simulink subsystem "LW_noaileron_dynamic"  (R2024b)
settings: Solver=VariableStepAuto  StartTime=0.0  StopTime=10.0  RelTol=1e-3
undefined symbols (not defined in the file or in its folder): decyear, DiscIntNeverNeededParam, Earth, F, Light, LW_ANGLE, MIL, ModelFailWind_ConstWindX, ModelFailWind_ConstWindY, ModelFailWind_ConstWindZ, ModelFailWind_GustWindFreq, ModelFailWind_GustWindStrength, ModelFailWind_isConstWind, ModelFailWind_isEnable, ModelFailWind_isGustWind, ModelFailWind_isSheerWind, ModelFailWind_isTurbWind, ModelInit_AngEuler, ModelInit_PosE, ModelInit_Rads, ModelInit_RateB, ModelInit_servoRads, ModelInit_VelB, ModelParam_DeltaRatemax, ModelParam_efficiency, ModelParam_envAltitude, ModelParam_LBb, ModelParam_LBc, ModelParam_LBClp, ModelParam_LBCmq, ModelParam_LBCnr, ModelParam_LBRho, ModelParam_LBS, ModelParam_lDeltamax, ModelParam_lDeltamin, ModelParam_motorp1, ModelParam_motorp2, ModelParam_motorp3, ModelParam_motorT, ModelParam_motorUp1, ModelParam_motorUp2, ModelParam_motorUp3, ModelParam_noiseFBa, ModelParam_noiseFBaSeed, ModelParam_noiseFNa, ModelParam_noiseFNaSeed, ModelParam_noiseMNa, ModelParam_noiseMNaSeed, ModelParam_rDeltamax, ModelParam_rDeltamin, ModelParam_servoT, ModelParam_temperature, ModelParam_uavCCm, ModelParam_uavCd, ModelParam_uavJ, ModelParam_uavMass, ModelParam_use_CoesaAtmosphereModel_density, ModelParam_use_CoesaAtmosphereModel_temperature, ModelReset_Euler, ModelReset_Pos ... (+5)
libraries: simulink x5, aerolibwind2 x3, sharedtransform x2, sharedutil x2, aerolibtransform2 x1, aerolibasang x1, aerolibatmos2 x1, aerolibconvert2 x1, aerolibgravity2 x1, shared6dof x1
(part 1 of 2)
settings Model: Creator=DELL  LastModifiedBy=bhcxq
settings SolverCC: AlgebraicLoopSolver=TrustRegion
settings DebuggingCC: UnconnectedInputMsg=warning  UnconnectedOutputMsg=warning  UnconnectedLineMsg=warning
settings ModelReferenceCC: EnableRefExpFcnMdlSchedulingChecks=on
settings RTWCC: GPUComputeCapability=3.5  DLArmComputeVersion=19.05

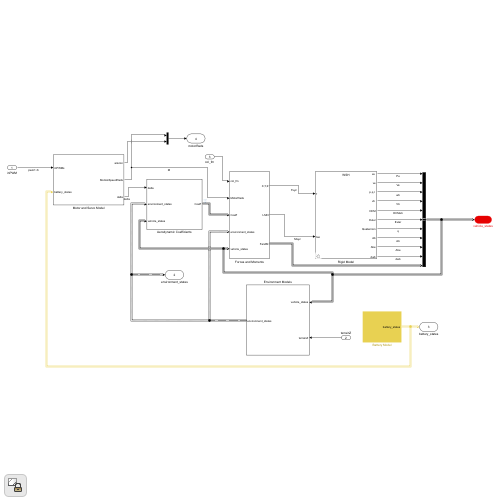
[thumbnail: Simulink's stored preview of the top-level diagram]
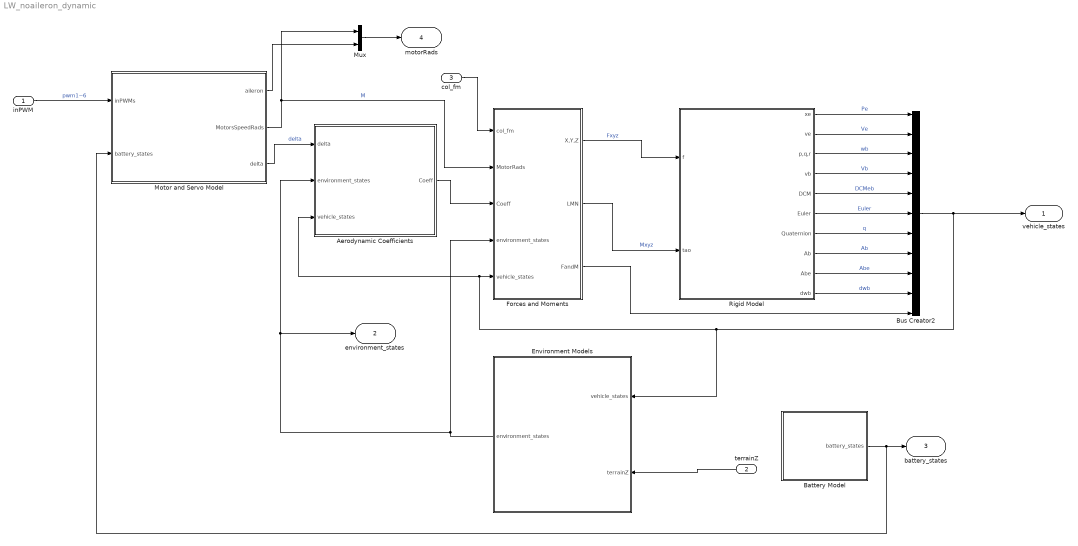
== system LW_noaileron_dynamic ==
  inPWM : Inport
  terrainZ : Inport  Port=2
  col_fm : Inport  Port=3
  Aerodynamic Coefficients : Subsystem
  Battery Model : Subsystem
  Bus Creator2 : BusCreator  Inputs=11
  Environment Models : Subsystem
  Forces and Moments : Subsystem
  Motor and Servo Model : Subsystem
  Mux : Mux  Inputs=2
  Rigid Model : Subsystem  Variant=on
  vehicle_states : Outport
  environment_states : Outport  Port=2
  battery_states : Outport  Port=3
  motorRads : Outport  Port=4
  wires:
  Rigid Model/5(DCM) -> Bus Creator2/5  "DCMeb"
  Rigid Model/9(Abe) -> Bus Creator2/9  "Abe"
  Rigid Model/4("vb ") -> Bus Creator2/4  "Vb"
  Rigid Model/2(ve) -> Bus Creator2/2  "Ve"
  Bus Creator2/1 -> Aerodynamic Coefficients/3(vehicle_states), Forces and Moments/5(vehicle_states), Environment Models/1(vehicle_states), vehicle_states/1
  Forces and Moments/1(X,Y,Z) -> Rigid Model/1(f)  "Fxyz"
  Rigid Model/1("xe ") -> Bus Creator2/1  "Pe"
  Forces and Moments/2(LMN) -> Rigid Model/2(tao)  "Mxyz"
  Rigid Model/6(Euler) -> Bus Creator2/6  "Euler"
  Aerodynamic Coefficients/1(Coeff) -> Forces and Moments/3(Coeff)
  Rigid Model/8(Ab) -> Bus Creator2/8  "Ab"
  inPWM/1 -> Motor and Servo Model/1(inPWMs)  "pwm1~6"
  Environment Models/1(environment_states) -> Aerodynamic Coefficients/2(environment_states), environment_states/1, Forces and Moments/4(environment_states)
  Rigid Model/3("p,q,r ") -> Bus Creator2/3  "wb"
  Motor and Servo Model/2(MotorsSpeedRads) -> Forces and Moments/2(MotorRads), Mux/1  "M"
  Mux/1 -> motorRads/1
  Motor and Servo Model/3(delta) -> Aerodynamic Coefficients/1(delta)  "delta"
  Rigid Model/7(Quaternion) -> Bus Creator2/7  "q"
  Battery Model/1(battery_states) -> battery_states/1, Motor and Servo Model/2(battery_states)
  Rigid Model/10(dwb) -> Bus Creator2/10  "dwb"
  terrainZ/1 -> Environment Models/2(terrainZ)
  Forces and Moments/3(FandM) -> Bus Creator2/11
  col_fm/1 -> Forces and Moments/1(col_fm)
  Motor and Servo Model/1(aileron) -> Mux/2

== system LW_noaileron_dynamic/Aerodynamic Coefficients ==
  delta : Inport
  environment_states : Inport  Port=2
  vehicle_states : Inport  Port=3
  Bus Creator : BusCreator  Inputs=6
  Bus Selector : BusSelector  OutputSignals=alpha,beta,airspeed  OutputAsBus=on
  Bus Selector1 : BusSelector  OutputSignals=wb  OutputAsBus=on
  aerodynamic coefficients : MATLAB Function  TreatAsAtomicUnit=on
  Coeff : Outport  VectorParamsAs1DForOutWhenUnconnected=off
  wires:
  aerodynamic coefficients/8(C_me) -> ?  "C_me"
  aerodynamic coefficients/7(C_m0) -> ?  "C_m0"
  environment_states/1 -> Bus Selector/1
  Bus Creator/1 -> Coeff/1
  aerodynamic coefficients/4(C_l) -> Bus Creator/4  "C_l"
  aerodynamic coefficients/5(C_m) -> Bus Creator/5  "C_m"
  aerodynamic coefficients/6(C_n) -> Bus Creator/6  "C_n"
  delta/1 -> aerodynamic coefficients/3(delta)
  Bus Selector/1 -> aerodynamic coefficients/1(incid)
  vehicle_states/1 -> Bus Selector1/1
  Bus Selector1/1 -> aerodynamic coefficients/2(wb)
  aerodynamic coefficients/1(C_D) -> Bus Creator/1  "C_D"
  aerodynamic coefficients/3(C_L) -> Bus Creator/3  "C_L"
  aerodynamic coefficients/2(C_Y) -> Bus Creator/2  "C_Y"

== system LW_noaileron_dynamic/Battery Model ==
  BatteryVol : Constant  Value=16
  Bus Creator : BusCreator  Inputs=2
  Constant : Constant  Value=4000
  battery_states : Outport
  wires:
  BatteryVol/1 -> Bus Creator/1  "Ub"
  Constant/1 -> Bus Creator/2  "RemCapa"
  Bus Creator/1 -> battery_states/1

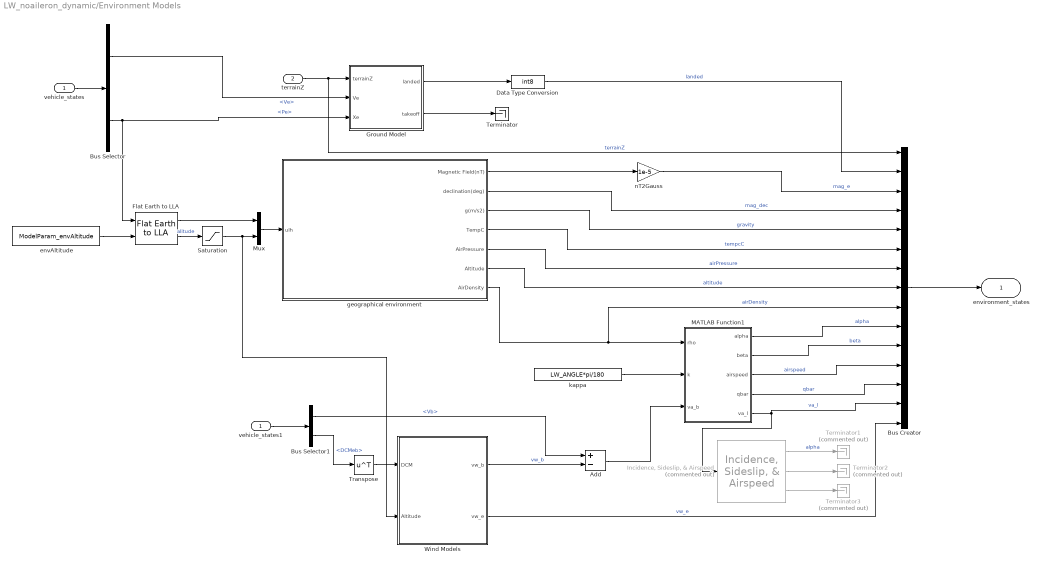
== system LW_noaileron_dynamic/Environment Models ==
  vehicle_states : Inport
  terrainZ : Inport  Port=2
  Add : Sum  Inputs=+-
  Bus Creator : BusCreator  Inputs=15  OutDataTypeStr=Bus: EnvironmentStates  NonVirtualBus=on
  Bus Selector : BusSelector  OutputSignals=Ve,Pe
  Bus Selector1 : BusSelector  OutputSignals=Vb,DCMeb
  Data Type Conversion : DataTypeConversion  OutDataTypeStr=int8  SaturateOnIntegerOverflow=off  RndMeth=Floor
  Flat Earth to LLA : aerolibtransform2/Flat Earth to LLA  units=Metric (MKS)  ptype=Earth (WGS84)  F=1/298.257223563  R=6378137  refPosPort=off  LL0=ModelParam_GPSLatLong  psi=0
  Ground Model : MATLAB Function  TreatAsAtomicUnit=on
  "Incidence, Sideslip, & Airspeed" : aerolibasang/Incidence, Sideslip, & Airspeed  Commented=on
  MATLAB Function1 : MATLAB Function  TreatAsAtomicUnit=on
  Mux : Mux  Inputs=2
  Saturation : Saturate  UpperLimit=10000  LowerLimit=0
  Terminator : Terminator
  Terminator1 : Terminator  Commented=on
  Terminator2 : Terminator  Commented=on
  Terminator3 : Terminator  Commented=on
  Transpose : Math  Operator=transpose  SignedPower=on
  Wind Models : Subsystem  TreatAsAtomicUnit=on
  envAltitude : Constant  Value=ModelParam_envAltitude
  geographical environment : Subsystem
  kappa : Constant  Value=LW_ANGLE*pi/180
  nT2Gauss : Gain  Gain=1e-5
  vehicle_states1 : InportShadow
  environment_states : Outport
  wires:
  MATLAB Function1/1(alpha) -> Bus Creator/10  "alpha"
  "Incidence, Sideslip, & Airspeed"/1 -> Terminator1/1  "alpha"
  "Incidence, Sideslip, & Airspeed"/3 -> Terminator3/1
  "Incidence, Sideslip, & Airspeed"/2 -> Terminator2/1
  MATLAB Function1/5(va_l) -> "Incidence, Sideslip, & Airspeed"/1, Bus Creator/14  "va_l"
  Flat Earth to LLA/2 -> Saturation/1  "alitude"
  vehicle_states/1 -> Bus Selector/1
  Bus Selector1/2 -> Transpose/1  "<DCMeb>"
  geographical environment/3(g(m/s2)) -> Bus Creator/5  "gravity"
  Mux/1 -> geographical environment/1(ulh)
  Flat Earth to LLA/1 -> Mux/1
  envAltitude/1 -> Flat Earth to LLA/2
  Transpose/1 -> Wind Models/1(DCM)
  geographical environment/1(Magnetic Field(nT)) -> nT2Gauss/1
  Bus Selector/2 -> Flat Earth to LLA/1, Ground Model/3(Xe)  "<Pe>"
  nT2Gauss/1 -> Bus Creator/3  "mag_e"
  geographical environment/2(declination(deg)) -> Bus Creator/4  "mag_dec"
  geographical environment/4(TempC) -> Bus Creator/6  "tempcC"
  geographical environment/5(AirPressure) -> Bus Creator/7  "airPressure"
  geographical environment/7(AirDensity) -> MATLAB Function1/1(rho), Bus Creator/9  "airDensity"
  Bus Creator/1 -> environment_states/1
  MATLAB Function1/2(beta) -> Bus Creator/11  "beta"
  MATLAB Function1/4(qbar) -> Bus Creator/13  "qbar"
  MATLAB Function1/3(airspeed) -> Bus Creator/12  "airspeed"
  Wind Models/1(vw_b) -> Add/2  "vw_b"
  kappa/1 -> MATLAB Function1/2(k)
  Bus Selector/1 -> Ground Model/2(Ve)  "<Ve>"
  Ground Model/2(takeoff) -> Terminator/1
  Ground Model/1(landed) -> Data Type Conversion/1
  terrainZ/1 -> Ground Model/1(terrainZ), Bus Creator/1  "terrainZ"
  Data Type Conversion/1 -> Bus Creator/2  "landed"
  Add/1 -> MATLAB Function1/3(va_b)
  Wind Models/2(vw_e) -> Bus Creator/15  "vw_e"
  vehicle_states1/1 -> Bus Selector1/1
  Bus Selector1/1 -> Add/1  "<Vb>"
  geographical environment/6(Altitude) -> Bus Creator/8  "altitude"
  Saturation/1 -> Wind Models/2(Altitude), Mux/2

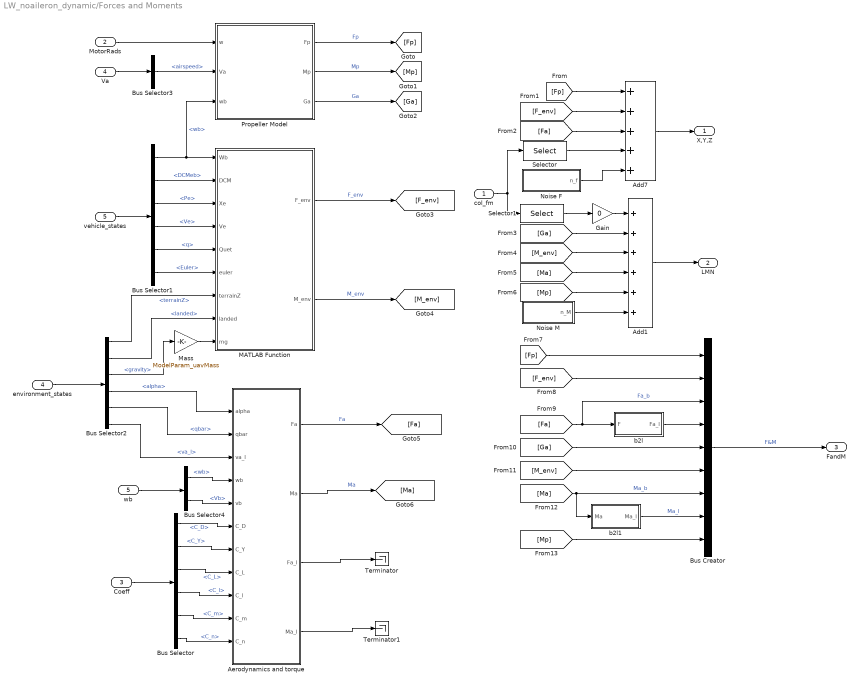
== system LW_noaileron_dynamic/Forces and Moments ==
  col_fm : Inport
  MotorRads : Inport  Port=2
  Coeff : Inport  Port=3
  environment_states : Inport  Port=4
  vehicle_states : Inport  Port=5
  Add1 : Sum  Inputs=++++++
  Add7 : Sum  Inputs=+++++
  Aerodynamics and torque : MATLAB Function  TreatAsAtomicUnit=on
  Bus Creator : BusCreator  Inputs=9
  Bus Selector : BusSelector  OutputSignals=C_D,C_Y,C_L,C_l,C_m,C_n
  Bus Selector1 : BusSelector  OutputSignals=wb,DCMeb,Pe,Ve,q,Euler
  Bus Selector2 : BusSelector  OutputSignals=terrainZ,landed,gravity,alpha,qbar,va_l
  Bus Selector3 : BusSelector  OutputSignals=airspeed
  Bus Selector4 : BusSelector  OutputSignals=wb,Vb
  Gain : Gain  Gain=0
  MATLAB Function : MATLAB Function  TreatAsAtomicUnit=on
  Mass : Gain  Gain=ModelParam_uavMass
  Noise F : Subsystem
  Noise M : Subsystem
  Propeller Model : MATLAB Function  TreatAsAtomicUnit=on
  Selector : Selector  InputPortWidth=6  IndexOptions=Index vector (dialog)  Indices=[1:3]  OutputSizes=1
  Selector1 : Selector  InputPortWidth=6  IndexOptions=Index vector (dialog)  Indices=[4:6]  OutputSizes=1
  Terminator : Terminator
  Terminator1 : Terminator
  Va : InportShadow  Port=4
  b2l : MATLAB Function  TreatAsAtomicUnit=on
  b2l1 : MATLAB Function  TreatAsAtomicUnit=on
  wb : InportShadow  Port=5
  X,Y,Z : Outport  PortDimensions=[3,1]  VectorParamsAs1DForOutWhenUnconnected=off
  LMN : Outport  Port=2  PortDimensions=[3,1]  VectorParamsAs1DForOutWhenUnconnected=off
  FandM : Outport  Port=3  VectorParamsAs1DForOutWhenUnconnected=off
  wires:
  Gain/1 -> Add1/1
  Noise M/1(n_M) -> Add1/6
  Noise F/1(n_f) -> Add7/5
  Aerodynamics and torque/4(Ma_l) -> Terminator1/1
  Aerodynamics and torque/3(Fa_l) -> Terminator/1
  b2l1/1(Ma_l) -> Bus Creator/8  "Ma_l"
  Selector1/1 -> Gain/1
  Selector/1 -> Add7/4
  col_fm/1 -> Selector1/1, Selector/1
  b2l/1(Fa_l) -> Bus Creator/4
  [Mp] -> Bus Creator/9
  [Ma] -> b2l1/1(Ma), Bus Creator/7  "Ma_b"
  [M_env] -> Bus Creator/6
  [Ga] -> Bus Creator/5
  [Fa] -> b2l/1(F), Bus Creator/3  "Fa_b"
  [F_env] -> Bus Creator/2
  [Fp] -> Bus Creator/1
  [Mp] -> Add1/5
  [Ma] -> Add1/4
  [M_env] -> Add1/3
  [Ga] -> Add1/2
  [Fa] -> Add7/3
  [F_env] -> Add7/2
  Aerodynamics and torque/2(Ma) -> [Ma]  "Ma"
  Aerodynamics and torque/1(Fa) -> [Fa]  "Fa"
  MATLAB Function/2(M_env) -> [M_env]  "M_env"
  [Fp] -> Add7/1
  Bus Creator/1 -> FandM/1  "F&M"
  Bus Selector2/2 -> MATLAB Function/8(landed)  "<landed>"
  Bus Selector1/6 -> MATLAB Function/6(euler)  "<Euler>"
  Bus Selector4/1 -> Aerodynamics and torque/4(wb)  "<wb>"
  Bus Selector2/6 -> Aerodynamics and torque/3(va_l)  "<va_l>"
  wb/1 -> Bus Selector4/1
  Bus Selector2/5 -> Aerodynamics and torque/2(qbar)  "<qbar>"
  Propeller Model/1(Fp) -> [Fp]  "Fp"
  Add7/1 -> X,Y,Z/1
  Propeller Model/2(Mp) -> [Mp]  "Mp"
  Add1/1 -> LMN/1
  environment_states/1 -> Bus Selector2/1
  Coeff/1 -> Bus Selector/1
  Bus Selector/1 -> Aerodynamics and torque/6(C_D)  "<C_D>"
  Bus Selector/2 -> Aerodynamics and torque/7(C_Y)  "<C_Y>"
  Bus Selector/3 -> Aerodynamics and torque/8(C_L)  "<C_L>"
  Bus Selector/4 -> Aerodynamics and torque/9(C_l)  "<C_l>"
  Bus Selector/5 -> Aerodynamics and torque/10(C_m)  "<C_m>"
  Bus Selector/6 -> Aerodynamics and torque/11(C_n)  "<C_n>"
  Propeller Model/3(Ga) -> [Ga]  "Ga"
  MotorRads/1 -> Propeller Model/1(w)
  Bus Selector3/1 -> Propeller Model/2(Va)  "<airspeed>"
  Bus Selector1/1 -> Propeller Model/3(wb), MATLAB Function/1(Wb)  "<wb>"
  Bus Selector1/5 -> MATLAB Function/5(Quet)  "<q>"
  Bus Selector1/3 -> MATLAB Function/3(Xe)  "<Pe>"
  Bus Selector2/1 -> MATLAB Function/7(terrainZ)  "<terrainZ>"
  Bus Selector1/2 -> MATLAB Function/2(DCM)  "<DCMeb>"
  MATLAB Function/1(F_env) -> [F_env]  "F_env"
  vehicle_states/1 -> Bus Selector1/1
  Bus Selector1/4 -> MATLAB Function/4(Ve)  "<Ve>"
  Bus Selector2/4 -> Aerodynamics and torque/1(alpha)  "<alpha>"
  Va/1 -> Bus Selector3/1
  Bus Selector2/3 -> Mass/1  "<gravity>"
  Mass/1 -> MATLAB Function/9(mg)
  Bus Selector4/2 -> Aerodynamics and torque/5(vb)  "<Vb>"

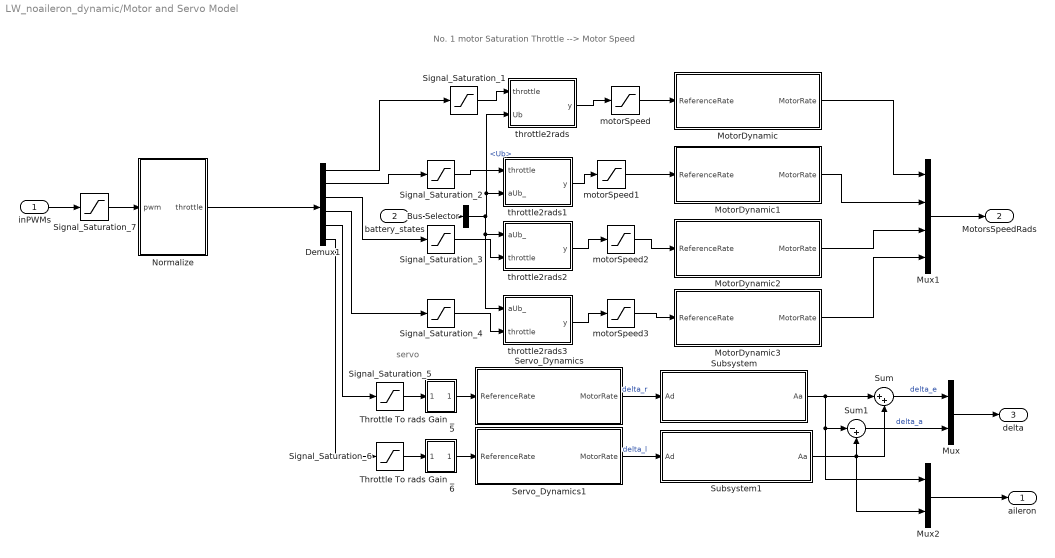
== system LW_noaileron_dynamic/Motor and Servo Model ==
  note: servo
  note: No. 1 motor
      |
      |          Saturation             Throttle --> Motor Speed
  inPWMs : Inport
  battery_states : Inport  Port=2
  Bus Selector : BusSelector  OutputSignals=Ub
  Demux1 : Demux  Outputs=6
  MotorDynamic : Subsystem  mask{motorT=ModelParam_motorT, Init_Rads=ModelInit_Rads}
      mask TypeOptions motorT: motorT/Value
      mask TypeOptions Init_Rads: Init_Rads/Value
      mask Display:
      | port_label('input', 1, '\varpi_{ss}(rad/s)', 'texmode', 'on');
      | port_label('output', 1, '\varpi(rad/s)', 'texmode', 'on');
  MotorDynamic1 : Subsystem  mask{motorT=ModelParam_motorT, Init_Rads=ModelInit_Rads}
      mask TypeOptions motorT: motorT/Value
      mask TypeOptions Init_Rads: Init_Rads/Value
      mask Display:
      | port_label('input', 1, '\varpi_{ss}(rad/s)', 'texmode', 'on');
      | port_label('output', 1, '\varpi(rad/s)', 'texmode', 'on');
  MotorDynamic2 : Subsystem  mask{motorT=ModelParam_motorT, Init_Rads=ModelInit_Rads}
      mask TypeOptions motorT: motorT/Value
      mask TypeOptions Init_Rads: Init_Rads/Value
      mask Display:
      | port_label('input', 1, '\varpi_{ss}(rad/s)', 'texmode', 'on');
      | port_label('output', 1, '\varpi(rad/s)', 'texmode', 'on');
  MotorDynamic3 : Subsystem  mask{motorT=ModelParam_motorT, Init_Rads=ModelInit_Rads}
      mask TypeOptions motorT: motorT/Value
      mask TypeOptions Init_Rads: Init_Rads/Value
      mask Display:
      | port_label('input', 1, '\varpi_{ss}(rad/s)', 'texmode', 'on');
      | port_label('output', 1, '\varpi(rad/s)', 'texmode', 'on');
  Mux : Mux  Inputs=2
  Mux1 : Mux
  Mux2 : Mux  Inputs=2
  Normalize : Subsystem
  Servo_Dynamics : Subsystem  mask{servoT=ModelParam_servoT, Init_Rads=ModelInit_servoRads}
      mask TypeOptions servoT: motorT/Value
      mask TypeOptions Init_Rads: Init_Rads/Value
      mask Display:
      | port_label('input', 1, '\theta_{ss}(rad/s)', 'texmode', 'on');
      | port_label('output', 1, '\theta(rad/s)', 'texmode', 'on');
  Servo_Dynamics1 : Subsystem  mask{servoT=ModelParam_servoT, Init_Rads=ModelInit_servoRads}
      mask TypeOptions servoT: motorT/Value
      mask TypeOptions Init_Rads: Init_Rads/Value
      mask Display:
      | port_label('input', 1, '\theta_{ss}(rad/s)', 'texmode', 'on');
      | port_label('output', 1, '\theta(rad/s)', 'texmode', 'on');
  Signal_Saturation_{1..4} (4 alike) : Saturate  UpperLimit=1  LowerLimit=0
  Signal_Saturation_5 : Saturate  UpperLimit=1  LowerLimit=-1
  Signal_Saturation_6 : Saturate  UpperLimit=1  LowerLimit=-1
  Signal_Saturation_7 : Saturate  UpperLimit=2000  LowerLimit=1000
  Subsystem : Subsystem  mask{DeltaRatemax=ModelParam_DeltaRatemax}
      mask prompts: DeltaRatemax "Simulink:blkprm_prompts:ConstConstValue"
      mask TypeOptions DeltaRatemax: Constant/Value
      mask DialogControl DeltaRatemax Prompt: 常量值:
      mask Display:
      | port_label('input', 1, 'Ad(rad/s)', 'texmode', 'on');
      | port_label('output', 1, 'Ac(rad/s)', 'texmode', 'on');
  Subsystem1 : Subsystem  mask{DeltaRatemax=ModelParam_DeltaRatemax}
      mask prompts: DeltaRatemax "Simulink:blkprm_prompts:ConstConstValue"
      mask TypeOptions DeltaRatemax: Constant/Value
      mask DialogControl DeltaRatemax Prompt: 常量值:
      mask Display:
      | port_label('input', 1, 'Ad(rad/s)', 'texmode', 'on');
      | port_label('output', 1, 'Ac(rad/s)', 'texmode', 'on');
  Sum : Sum  Inputs=|++
  Sum1 : Sum  Inputs=|-+
  Throttle To rads Gain _5 : Subsystem
  Throttle To rads Gain _6 : Subsystem
  motorSpeed{,1..3} (4 alike) : Saturate  UpperLimit=9000  LowerLimit=0
  throttle2rads : MATLAB Function  TreatAsAtomicUnit=on
  throttle2rads1 : MATLAB Function  TreatAsAtomicUnit=on
  throttle2rads2 : MATLAB Function  TreatAsAtomicUnit=on
  throttle2rads3 : MATLAB Function  TreatAsAtomicUnit=on
  aileron : Outport  PortDimensions=2  VectorParamsAs1DForOutWhenUnconnected=off
  MotorsSpeedRads : Outport  Port=2  PortDimensions=4  VectorParamsAs1DForOutWhenUnconnected=off
  delta : Outport  Port=3  PortDimensions=2  VectorParamsAs1DForOutWhenUnconnected=off
  wires:
  Bus Selector/1 -> throttle2rads1/2(aUb_), throttle2rads/2(Ub), throttle2rads2/1(aUb_), throttle2rads3/1(aUb_)  "<Ub>"
  battery_states/1 -> Bus Selector/1
  Mux2/1 -> aileron/1
  Subsystem1/1(Aa) -> Sum/2, Sum1/2, Mux2/2
  Subsystem/1(Aa) -> Mux2/1, Sum1/1, Sum/1
  motorSpeed3/1 -> MotorDynamic3/1(ReferenceRate)
  Signal_Saturation_4/1 -> throttle2rads3/2(throttle)
  Signal_Saturation_3/1 -> throttle2rads2/2(throttle)
  Signal_Saturation_2/1 -> throttle2rads1/1(throttle)
  MotorDynamic3/1(MotorRate) -> Mux1/4
  MotorDynamic2/1(MotorRate) -> Mux1/3
  MotorDynamic1/1(MotorRate) -> Mux1/2
  Signal_Saturation_1/1 -> throttle2rads/1(throttle)
  Mux1/1 -> MotorsSpeedRads/1
  motorSpeed2/1 -> MotorDynamic2/1(ReferenceRate)
  motorSpeed1/1 -> MotorDynamic1/1(ReferenceRate)
  throttle2rads/1(y) -> motorSpeed/1
  Demux1/3 -> Signal_Saturation_3/1
  Demux1/2 -> Signal_Saturation_2/1
  Demux1/1 -> Signal_Saturation_1/1
  Signal_Saturation_5/1 -> Throttle To rads Gain _5/1(In5)
  Throttle To rads Gain _5/1(Out5) -> Servo_Dynamics/1(ReferenceRate)
  Mux/1 -> delta/1
  Throttle To rads Gain _6/1(Out5) -> Servo_Dynamics1/1(ReferenceRate)
  Signal_Saturation_6/1 -> Throttle To rads Gain _6/1(In5)
  Demux1/4 -> Signal_Saturation_4/1
  Servo_Dynamics/1(MotorRate) -> Subsystem/1(Ad)  "delta_r"
  Servo_Dynamics1/1(MotorRate) -> Subsystem1/1(Ad)  "delta_l"
  Sum/1 -> Mux/1  "delta_e"
  Sum1/1 -> Mux/2  "delta_a"
  Demux1/5 -> Signal_Saturation_5/1
  Demux1/6 -> Signal_Saturation_6/1
  inPWMs/1 -> Signal_Saturation_7/1
  Normalize/1(throttle) -> Demux1/1
  MotorDynamic/1(MotorRate) -> Mux1/1
  motorSpeed/1 -> MotorDynamic/1(ReferenceRate)
  throttle2rads1/1(y) -> motorSpeed1/1
  throttle2rads2/1(y) -> motorSpeed2/1
  throttle2rads3/1(y) -> motorSpeed3/1
  Signal_Saturation_7/1 -> Normalize/1(pwm)

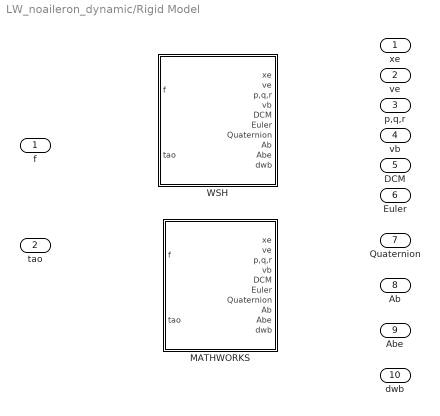
== system LW_noaileron_dynamic/Rigid Model ==
  f : Inport  PortDimensions=[3,1]
  tao : Inport  Port=2  PortDimensions=[3,1]
  MATHWORKS : Subsystem  VariantControl=VSS_6DOF_MATHWORKS
  WSH : Subsystem  VariantControl=VSS_6DOF_WSH
  "xe " : Outport  VectorParamsAs1DForOutWhenUnconnected=off
  ve : Outport  Port=2  VectorParamsAs1DForOutWhenUnconnected=off
  "p,q,r " : Outport  Port=3  VectorParamsAs1DForOutWhenUnconnected=off
  "vb " : Outport  Port=4  VectorParamsAs1DForOutWhenUnconnected=off
  DCM : Outport  Port=5  VectorParamsAs1DForOutWhenUnconnected=off
  Euler : Outport  Port=6  VectorParamsAs1DForOutWhenUnconnected=off
  Quaternion : Outport  Port=7  VectorParamsAs1DForOutWhenUnconnected=off
  Ab : Outport  Port=8  VectorParamsAs1DForOutWhenUnconnected=off
  Abe : Outport  Port=9  VectorParamsAs1DForOutWhenUnconnected=off
  dwb : Outport  Port=10  VectorParamsAs1DForOutWhenUnconnected=off

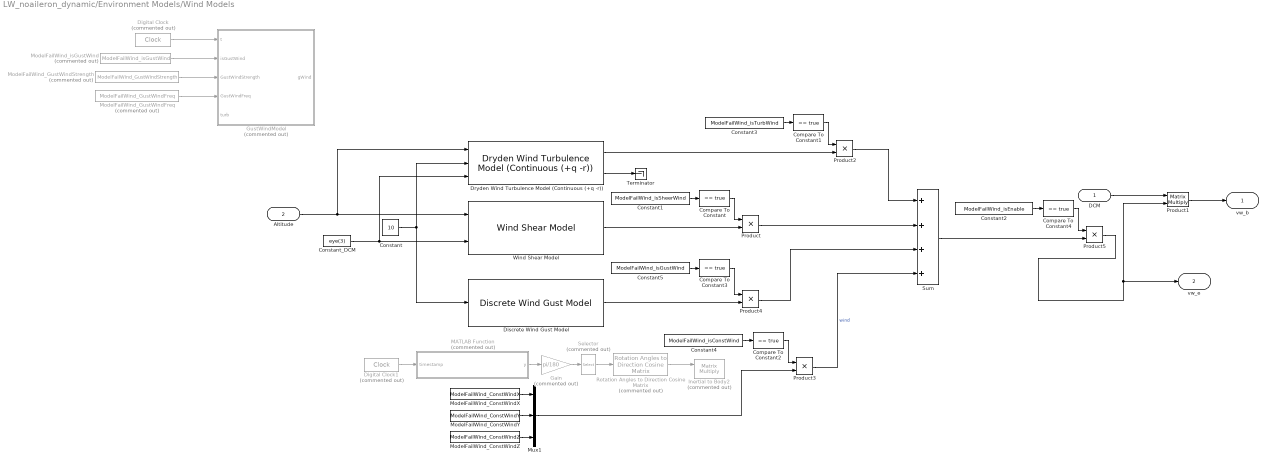
== system LW_noaileron_dynamic/Environment Models/Wind Models ==
  DCM : Inport
  Altitude : Inport  Port=2
  Compare To Constant{,1..4} (5 alike) : simulink/Logic and Bit Operations/Compare To Constant  relop===  const=true  OutDataTypeStr=uint8
  Constant : Constant  Value=10
  Constant1 : Constant  Value=ModelFailWind_isSheerWind
  Constant2 : Constant  Value=ModelFailWind_isEnable
  Constant3 : Constant  Value=ModelFailWind_isTurbWind
  Constant4 : Constant  Value=ModelFailWind_isConstWind
  Constant5 : Constant  Value=ModelFailWind_isGustWind
  Constant_DCM : Constant  Value=eye(3)
  Digital Clock : DigitalClock  Commented=on  SampleTime=SampleTime
  Digital Clock1 : DigitalClock  Commented=on  SampleTime=0.001
  Discrete Wind Gust Model : aerolibwind2/Discrete Wind Gust Model  units=Metric (MKS)  Gx=on  Gy=on  Gz=on  t_0=ModelFailWind_GustStartTime  d_m=[120 120 80]  v_m=ModelFailWind_GustWindAmplitude
  Dryden Wind Turbulence Model (Continuous (+q -r)) : aerolibwind2/Dryden Wind Turbulence Model  (Continuous (+q -r))  units=Metric (MKS)  spec=MIL-F-8785C  model=Continuous Dryden (+q -r)  W20=10  Wdeg=0  TurbProb=10^-2 - Light  L_high=533.4  Wingspan=1  ts=0.001  Seed=[23341 23342 23343 23344]  T_on=on
  Gain : Gain  Commented=on  Gain=pi/180
  GustWindModel : MATLAB Function  Commented=on  TreatAsAtomicUnit=on
  Inertial to Body2 : Product  Commented=on  Multiplication=Matrix(*)  InputSameDT=on  SaturateOnIntegerOverflow=on  OutDataTypeStr=Inherit: Same as first input
  MATLAB Function : MATLAB Function  Commented=on  TreatAsAtomicUnit=on
  ModelFailWind_ConstWindX : Constant  Value=ModelFailWind_ConstWindX
  ModelFailWind_ConstWindY : Constant  Value=ModelFailWind_ConstWindY
  ModelFailWind_ConstWindZ : Constant  Value=ModelFailWind_ConstWindZ
  ModelFailWind_GustWindFreq : Constant  Commented=on  Value=ModelFailWind_GustWindFreq
  ModelFailWind_GustWindStrength : Constant  Commented=on  Value=ModelFailWind_GustWindStrength
  ModelFailWind_isGustWind : Constant  Commented=on  Value=ModelFailWind_isGustWind
  Mux1 : Mux  Inputs=3
  Product{,2..5} (5 alike) : Product
  Product1 : Product  Multiplication=Matrix(*)
  Rotation Angles to Direction Cosine Matrix : sharedtransform/Rotation Angles to Direction Cosine Matrix  Commented=on  rotationOrder=ZYX  aMode=aMode
  Selector : Selector  Commented=on  InputPortWidth=3  IndexOptions=Index vector (dialog)  Indices=[3 2 1]  OutputSizes=1
  Sum : Sum  Inputs=++++
  Terminator : Terminator
  Wind Shear Model : aerolibwind2/Wind Shear Model  units=Metric (MKS)  phase=Category C - Terminal Flight Phase  W_20=15  Wdeg=0
  vw_b : Outport  VectorParamsAs1DForOutWhenUnconnected=off
  vw_e : Outport  Port=2  VectorParamsAs1DForOutWhenUnconnected=off
  wires:
  Product5/1 -> vw_e/1, Product1/2
  Sum/1 -> Product5/2
  Constant2/1 -> Compare To Constant4/1
  Compare To Constant4/1 -> Product5/1
  ModelFailWind_ConstWindZ/1 -> Mux1/3
  Digital Clock1/1 -> MATLAB Function/1(timestamp)
  Constant_DCM/1 -> Dryden Wind Turbulence Model (Continuous (+q -r))/3, Wind Shear Model/2
  Wind Shear Model/1 -> Product/2
  Product4/1 -> Sum/3
  Dryden Wind Turbulence Model (Continuous (+q -r))/2 -> Terminator/1
  Constant/1 -> Dryden Wind Turbulence Model (Continuous (+q -r))/2, Discrete Wind Gust Model/1
  Altitude/1 -> Dryden Wind Turbulence Model (Continuous (+q -r))/1, Wind Shear Model/1
  ModelFailWind_GustWindFreq/1 -> GustWindModel/4(GustWindFreq)
  ModelFailWind_isGustWind/1 -> GustWindModel/2(isGustWind)
  ModelFailWind_GustWindStrength/1 -> GustWindModel/3(GustWindStrength)
  Digital Clock/1 -> GustWindModel/1(t)
  Product2/1 -> Sum/1
  ModelFailWind_ConstWindY/1 -> Mux1/2
  ModelFailWind_ConstWindX/1 -> Mux1/1
  Constant1/1 -> Compare To Constant/1
  Compare To Constant/1 -> Product/1
  Product/1 -> Sum/2
  DCM/1 -> Product1/1
  Product1/1 -> vw_b/1
  MATLAB Function/1(y) -> Gain/1
  Selector/1 -> Rotation Angles to Direction Cosine Matrix/1
  Rotation Angles to Direction Cosine Matrix/1 -> Inertial to Body2/1
  Gain/1 -> Selector/1
  Product3/1 -> Sum/4  "wind"
  Compare To Constant1/1 -> Product2/1
  Constant3/1 -> Compare To Constant1/1
  Dryden Wind Turbulence Model (Continuous (+q -r))/1 -> Product2/2
  Compare To Constant2/1 -> Product3/1
  Constant4/1 -> Compare To Constant2/1
  Mux1/1 -> Product3/2
  Compare To Constant3/1 -> Product4/1
  Constant5/1 -> Compare To Constant3/1
  Discrete Wind Gust Model/1 -> Product4/2

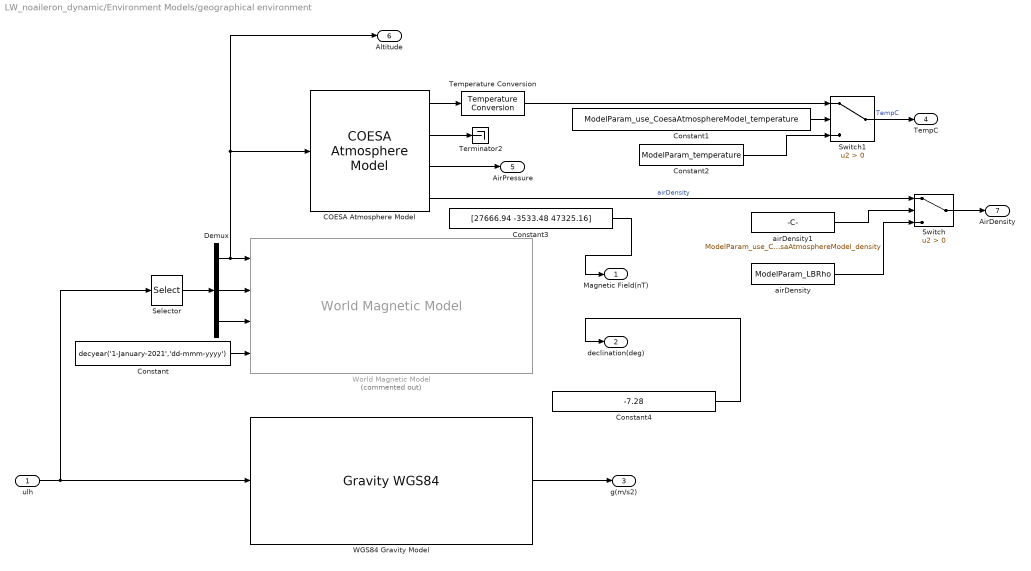
== system LW_noaileron_dynamic/Environment Models/geographical environment ==
  ulh : Inport
  COESA Atmosphere Model : aerolibatmos2/COESA Atmosphere Model  units=Metric (MKS)  spec=1976 COESA-extended U.S. Standard Atmosphere  model=Profile  profile_var=High temperature  profile_percent=1%  profile_alt=5 km (16404 ft)  envelope_var=High temperature  envelope_percent=1%  action=Warning
  Constant : Constant  Value=decyear('1-January-2021','dd-mmm-yyyy')
  Constant1 : Constant  Value=ModelParam_use_CoesaAtmosphereModel_temperature
  Constant2 : Constant  Value=ModelParam_temperature
  Constant3 : Constant  Value=[27666.94 -3533.48 47325.16]
  Constant4 : Constant  Value=-7.28
  Demux : Demux  Outputs=3
  Selector : Selector  InputPortWidth=3  IndexOptions=Index vector (dialog)  Indices=[3 1 2]  OutputSizes=1
  Switch : Switch  Criteria=u2 > Threshold  SaturateOnIntegerOverflow=off  InputSameDT=off
  Switch1 : Switch  Criteria=u2 > Threshold  SaturateOnIntegerOverflow=off  InputSameDT=off
  Temperature Conversion : aerolibconvert2/Temperature Conversion  IU=K  OU=C
  Terminator2 : Terminator
  "WGS84 Gravity Model  " : GravityWGS84
  World Magnetic Model : aerolibgravity2/World Magnetic Model  Commented=on  model=WMM2020 (2020-2025)  customFile='WMM2020.COF'  units=Metric (MKS)  time_in=on  month=January  day=1  year=2020  action=Error  h_out=off  dec_out=on  inc_out=off  ti_out=off
  airDensity : Constant  Value=ModelParam_LBRho
  airDensity1 : Constant  Value=ModelParam_use_CoesaAtmosphereModel_density
  Magnetic Field(nT) : Outport
  declination(deg) : Outport  Port=2
  g(m/s2) : Outport  Port=3
  TempC : Outport  Port=4
  AirPressure : Outport  Port=5
  Altitude : Outport  Port=6
  AirDensity : Outport  Port=7
  wires:
  Constant4/1 -> declination(deg)/1
  Constant3/1 -> Magnetic Field(nT)/1
  Switch/1 -> AirDensity/1
  COESA Atmosphere Model/3 -> AirPressure/1
  COESA Atmosphere Model/2 -> Terminator2/1
  "WGS84 Gravity Model  "/1 -> g(m/s2)/1
  ulh/1 -> "WGS84 Gravity Model  "/1, Selector/1
  Selector/1 -> Demux/1
  Demux/1 -> Altitude/1, COESA Atmosphere Model/1, World Magnetic Model/1
  Demux/2 -> World Magnetic Model/2
  Demux/3 -> World Magnetic Model/3
  Constant/1 -> World Magnetic Model/4
  Temperature Conversion/1 -> Switch1/1
  Constant2/1 -> Switch1/3
  Constant1/1 -> Switch1/2
  Switch1/1 -> TempC/1  "TempC"
  COESA Atmosphere Model/1 -> Temperature Conversion/1
  airDensity1/1 -> Switch/2
  airDensity/1 -> Switch/3
  COESA Atmosphere Model/4 -> Switch/1  "airDensity"

== system LW_noaileron_dynamic/Forces and Moments/Noise F ==
  Add : Sum
  Demux : Demux  Outputs=3
  Integrator : Integrator
  Mux : Mux  Inputs=3
  Random Number : RandomNumber  Variance=ModelParam_noiseFNa  Seed=ModelParam_noiseFNaSeed  SampleTime=0.004
  Random Number1 : RandomNumber  Variance=ModelParam_noiseFBa  Seed=ModelParam_noiseFBaSeed  SampleTime=0.004
  Transfer Fcn : TransferFcn  Denominator=[0.1 1]
  Transfer Fcn1 : TransferFcn  Denominator=[0.1 1]
  Transfer Fcn2 : TransferFcn  Denominator=[0.1 1]
  n_f : Outport
  wires:
  Mux/1 -> n_f/1
  Random Number1/1 -> Integrator/1
  Demux/3 -> Transfer Fcn2/1
  Random Number/1 -> Add/1
  Transfer Fcn/1 -> Mux/1
  Integrator/1 -> Add/2
  Add/1 -> Demux/1
  Transfer Fcn1/1 -> Mux/2
  Demux/2 -> Transfer Fcn1/1
  Transfer Fcn2/1 -> Mux/3
  Demux/1 -> Transfer Fcn/1

== system LW_noaileron_dynamic/Forces and Moments/Noise M ==
  Add2 : Sum
  Demux1 : Demux  Outputs=3
  Integrator1 : Integrator
  Mux1 : Mux  Inputs=3
  Random Number2 : RandomNumber  Variance=ModelParam_noiseMNa  Seed=ModelParam_noiseMNaSeed  SampleTime=0.004
  Random Number3 : RandomNumber  Variance=ModelParam_noiseFBa  Seed=ModelParam_noiseFBaSeed  SampleTime=0.004
  Transfer Fcn3 : TransferFcn  Denominator=[0.1 1]
  Transfer Fcn4 : TransferFcn  Denominator=[0.1 1]
  Transfer Fcn5 : TransferFcn  Denominator=[0.1 1]
  n_M : Outport
  wires:
  Mux1/1 -> n_M/1
  Random Number3/1 -> Integrator1/1
  Random Number2/1 -> Add2/1
  Add2/1 -> Demux1/1
  Transfer Fcn4/1 -> Mux1/2
  Transfer Fcn5/1 -> Mux1/3
  Demux1/1 -> Transfer Fcn3/1
  Demux1/3 -> Transfer Fcn5/1
  Integrator1/1 -> Add2/2
  Transfer Fcn3/1 -> Mux1/1
  Demux1/2 -> Transfer Fcn4/1

== system LW_noaileron_dynamic/Motor and Servo Model/MotorDynamic ==
  note: Motor Dynamic
      | w=1/(Ts+1)*wb
  ReferenceRate : Inport  Unit=rad/s
  Discrete-Time Integrator : DiscreteIntegrator  InitialConditionSource=external  InitialCondition=ModelInit_Rads  SampleTime=-1  ICPrevOutput=DiscIntNeverNeededParam  ICPrevScaledInput=DiscIntNeverNeededParam
  Divide : Product  Inputs=*/
  Init_Rads : Constant  Value=Init_Rads
  Sum : Sum  Inputs=-+|
  motorT : Constant  Value=motorT
  MotorRate : Outport  Unit=rad/s
  wires:
  Discrete-Time Integrator/1 -> MotorRate/1, Sum/1
  Divide/1 -> Discrete-Time Integrator/1
  motorT/1 -> Divide/2
  Sum/1 -> Divide/1
  ReferenceRate/1 -> Sum/2
  Init_Rads/1 -> Discrete-Time Integrator/2

== system LW_noaileron_dynamic/Motor and Servo Model/MotorDynamic1 ==
  note: Motor Dynamic
      | w=1/(Ts+1)*wb
  ReferenceRate : Inport  Unit=rad/s
  Discrete-Time Integrator : DiscreteIntegrator  InitialConditionSource=external  InitialCondition=ModelInit_Rads  SampleTime=-1  ICPrevOutput=DiscIntNeverNeededParam  ICPrevScaledInput=DiscIntNeverNeededParam
  Divide : Product  Inputs=*/
  Init_Rads : Constant  Value=Init_Rads
  Sum : Sum  Inputs=-+|
  motorT : Constant  Value=motorT
  MotorRate : Outport  Unit=rad/s
  wires:
  Init_Rads/1 -> Discrete-Time Integrator/2
  ReferenceRate/1 -> Sum/2
  Sum/1 -> Divide/1
  motorT/1 -> Divide/2
  Divide/1 -> Discrete-Time Integrator/1
  Discrete-Time Integrator/1 -> Sum/1, MotorRate/1

== system LW_noaileron_dynamic/Motor and Servo Model/MotorDynamic2 ==
  note: Motor Dynamic
      | w=1/(Ts+1)*wb
  ReferenceRate : Inport  Unit=rad/s
  Discrete-Time Integrator : DiscreteIntegrator  InitialConditionSource=external  InitialCondition=ModelInit_Rads  SampleTime=-1  ICPrevOutput=DiscIntNeverNeededParam  ICPrevScaledInput=DiscIntNeverNeededParam
  Divide : Product  Inputs=*/
  Init_Rads : Constant  Value=Init_Rads
  Sum : Sum  Inputs=-+|
  motorT : Constant  Value=motorT
  MotorRate : Outport  Unit=rad/s
  wires:
  Discrete-Time Integrator/1 -> MotorRate/1, Sum/1
  Divide/1 -> Discrete-Time Integrator/1
  motorT/1 -> Divide/2
  Sum/1 -> Divide/1
  ReferenceRate/1 -> Sum/2
  Init_Rads/1 -> Discrete-Time Integrator/2

== system LW_noaileron_dynamic/Motor and Servo Model/MotorDynamic3 ==
  note: Motor Dynamic
      | w=1/(Ts+1)*wb
  ReferenceRate : Inport  Unit=rad/s
  Discrete-Time Integrator : DiscreteIntegrator  InitialConditionSource=external  InitialCondition=ModelInit_Rads  SampleTime=-1  ICPrevOutput=DiscIntNeverNeededParam  ICPrevScaledInput=DiscIntNeverNeededParam
  Divide : Product  Inputs=*/
  Init_Rads : Constant  Value=Init_Rads
  Sum : Sum  Inputs=-+|
  motorT : Constant  Value=motorT
  MotorRate : Outport  Unit=rad/s
  wires:
  Init_Rads/1 -> Discrete-Time Integrator/2
  ReferenceRate/1 -> Sum/2
  Sum/1 -> Divide/1
  motorT/1 -> Divide/2
  Divide/1 -> Discrete-Time Integrator/1
  Discrete-Time Integrator/1 -> Sum/1, MotorRate/1

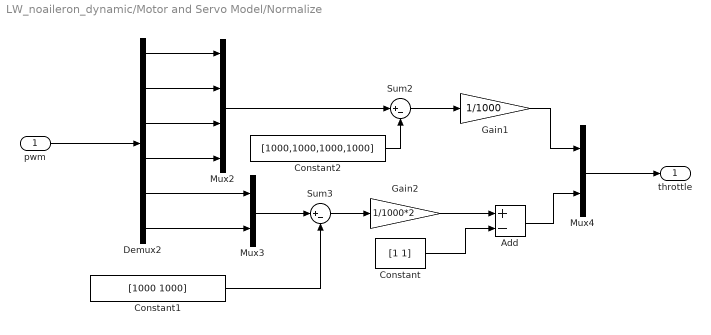
== system LW_noaileron_dynamic/Motor and Servo Model/Normalize ==
  pwm : Inport
  Add : Sum  Inputs=+-
  Constant : Constant  Value=[1 1]
  Constant1 : Constant  Value=[1000 1000]
  Constant2 : Constant  Value=[1000,1000,1000,1000]
  Demux2 : Demux  Outputs=6
  Gain1 : Gain  Gain=1/1000
  Gain2 : Gain  Gain=1/1000*2
  Mux2 : Mux
  Mux3 : Mux  Inputs=2
  Mux4 : Mux  Inputs=2
  Sum2 : Sum  Inputs=|+-
  Sum3 : Sum  Inputs=|+-
  throttle : Outport  VectorParamsAs1DForOutWhenUnconnected=off
  wires:
  Gain1/1 -> Mux4/1
  Constant2/1 -> Sum2/2
  Sum2/1 -> Gain1/1
  Mux2/1 -> Sum2/1
  pwm/1 -> Demux2/1
  Demux2/1 -> Mux2/1
  Demux2/2 -> Mux2/2
  Demux2/5 -> Mux3/1
  Mux4/1 -> throttle/1
  Demux2/6 -> Mux3/2
  Gain2/1 -> Add/1
  Demux2/3 -> Mux2/3
  Mux3/1 -> Sum3/1
  Sum3/1 -> Gain2/1
  Demux2/4 -> Mux2/4
  Constant1/1 -> Sum3/2
  Add/1 -> Mux4/2
  Constant/1 -> Add/2

== system LW_noaileron_dynamic/Motor and Servo Model/Servo_Dynamics ==
  note: Motor Dynamic
      | w=1/(Ts+1)*wb
  ReferenceRate : Inport  Unit=rad/s
  Discrete-Time Integrator : DiscreteIntegrator  InitialConditionSource=external  InitialCondition=ModelInit_Rads  SampleTime=-1  ICPrevOutput=DiscIntNeverNeededParam  ICPrevScaledInput=DiscIntNeverNeededParam
  Divide : Product  Inputs=*/
  Init_Rads : Constant  Value=Init_Rads
  Sum : Sum  Inputs=-+|
  motorT : Constant  Value=servoT
  MotorRate : Outport  Unit=rad/s
  wires:
  Discrete-Time Integrator/1 -> MotorRate/1, Sum/1
  Divide/1 -> Discrete-Time Integrator/1
  motorT/1 -> Divide/2
  Sum/1 -> Divide/1
  ReferenceRate/1 -> Sum/2
  Init_Rads/1 -> Discrete-Time Integrator/2

== system LW_noaileron_dynamic/Motor and Servo Model/Servo_Dynamics1 ==
  note: Motor Dynamic
      | w=1/(Ts+1)*wb
  ReferenceRate : Inport  Unit=rad/s
  Discrete-Time Integrator : DiscreteIntegrator  InitialConditionSource=external  InitialCondition=ModelInit_Rads  SampleTime=-1  ICPrevOutput=DiscIntNeverNeededParam  ICPrevScaledInput=DiscIntNeverNeededParam
  Divide : Product  Inputs=*/
  Init_Rads : Constant  Value=Init_Rads
  Sum : Sum  Inputs=-+|
  motorT : Constant  Value=servoT
  MotorRate : Outport  Unit=rad/s
  wires:
  Init_Rads/1 -> Discrete-Time Integrator/2
  ReferenceRate/1 -> Sum/2
  Sum/1 -> Divide/1
  motorT/1 -> Divide/2
  Divide/1 -> Discrete-Time Integrator/1
  Discrete-Time Integrator/1 -> Sum/1, MotorRate/1

== system LW_noaileron_dynamic/Motor and Servo Model/Subsystem ==
  Ad : Inport
  Add : Sum  Inputs=+-
  Constant : Constant  Value=DeltaRatemax
  Digital Clock : DigitalClock  SampleTime=0.001
  MATLAB Function : MATLAB Function  TreatAsAtomicUnit=on
  Unit Delay : UnitDelay  SampleTime=-1  HasFrameUpgradeWarning=on
  Aa : Outport
  wires:
  Ad/1 -> MATLAB Function/1(Ad)
  Add/1 -> MATLAB Function/2(dt)
  Constant/1 -> MATLAB Function/3(rate_max)
  Digital Clock/1 -> Unit Delay/1, Add/1
  Unit Delay/1 -> Add/2
  MATLAB Function/1(Aa) -> Aa/1

== system LW_noaileron_dynamic/Motor and Servo Model/Subsystem1 ==
  Ad : Inport
  Add : Sum  Inputs=+-
  Constant : Constant  Value=DeltaRatemax
  Digital Clock : DigitalClock  SampleTime=0.001
  MATLAB Function : MATLAB Function  TreatAsAtomicUnit=on
  Unit Delay : UnitDelay  SampleTime=-1  HasFrameUpgradeWarning=on
  Aa : Outport
  wires:
  MATLAB Function/1(Aa) -> Aa/1
  Unit Delay/1 -> Add/2
  Digital Clock/1 -> Add/1, Unit Delay/1
  Constant/1 -> MATLAB Function/3(rate_max)
  Add/1 -> MATLAB Function/2(dt)
  Ad/1 -> MATLAB Function/1(Ad)

== system LW_noaileron_dynamic/Motor and Servo Model/Throttle To rads Gain _5 ==
  In5 : Inport
  Constant : Constant  Value=ModelParam_rDeltamax
  Constant1 : Constant  Value=-ModelParam_rDeltamin
  Product : Product
  Switch : Switch  Criteria=u2 > Threshold  SaturateOnIntegerOverflow=off  InputSameDT=off
  Out5 : Outport  VectorParamsAs1DForOutWhenUnconnected=off
  wires:
  Constant1/1 -> Switch/3
  Switch/1 -> Product/1
  Constant/1 -> Switch/1
  In5/1 -> Switch/2, Product/2
  Product/1 -> Out5/1

== system LW_noaileron_dynamic/Motor and Servo Model/Throttle To rads Gain _6 ==
  In5 : Inport
  Constant : Constant  Value=ModelParam_lDeltamax
  Constant1 : Constant  Value=-ModelParam_lDeltamin
  Product : Product
  Switch : Switch  Criteria=u2 > Threshold  SaturateOnIntegerOverflow=off  InputSameDT=off
  Out5 : Outport  VectorParamsAs1DForOutWhenUnconnected=off
  wires:
  In5/1 -> Switch/2, Product/2
  Constant/1 -> Switch/1
  Constant1/1 -> Switch/3
  Switch/1 -> Product/1
  Product/1 -> Out5/1

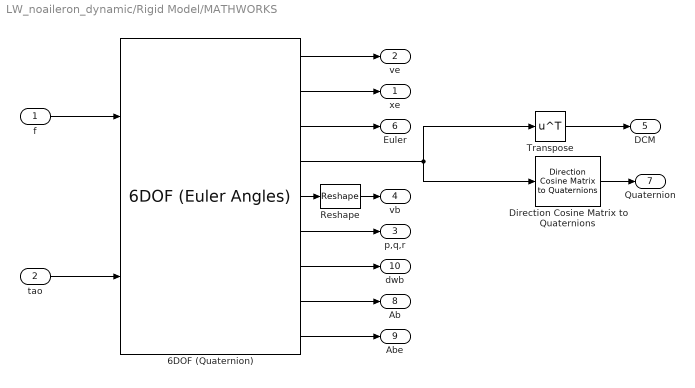
== system LW_noaileron_dynamic/Rigid Model/MATHWORKS ==
  f : Inport
  tao : Inport  Port=2
  6DOF (Quaternion) : shared6dof/6DOF (Euler Angles)  units=Metric (MKS)  mtype=Fixed  rep=Quaternion  xme_0=ModelInit_PosE  Vm_0=ModelInit_VelB  eul_0=ModelInit_AngEuler  pm_0=ModelInit_RateB  mass_0=ModelParam_uavMass  mass_e=0.5  mass_f=2.0  inertia=ModelParam_uavJ  inertia_e=eye(3)  inertia_f=2*eye(3)  k_quat=1.0  vre_flag=on  abi_flag=on  aMode=aMode  xme_statename=''  Vm_statename=''  eul_statename=''  quat_statename=''  pm_statename=''  mass_statename=''
  Direction Cosine Matrix to Quaternions : sharedtransform/Direction Cosine Matrix  to Quaternions  aMode=0  action=None  tolerance=eps(2)
  Reshape : Reshape  OutputDimensionality=Column vector (2-D)
  Transpose : Math  Operator=transpose  SignedPower=on
  "xe " : Outport  PortDimensions=[3,1]  VectorParamsAs1DForOutWhenUnconnected=off
  ve : Outport  Port=2  PortDimensions=[3,1]  VectorParamsAs1DForOutWhenUnconnected=off
  "p,q,r " : Outport  Port=3  PortDimensions=[3,1]  VectorParamsAs1DForOutWhenUnconnected=off
  "vb " : Outport  Port=4  PortDimensions=[3,1]  VectorParamsAs1DForOutWhenUnconnected=off
  DCM : Outport  Port=5  VectorParamsAs1DForOutWhenUnconnected=off
  Euler : Outport  Port=6  PortDimensions=[3,1]  VectorParamsAs1DForOutWhenUnconnected=off
  Quaternion : Outport  Port=7  VectorParamsAs1DForOutWhenUnconnected=off
  Ab : Outport  Port=8  PortDimensions=[3,1]  VectorParamsAs1DForOutWhenUnconnected=off
  Abe : Outport  Port=9  PortDimensions=[3,1]  VectorParamsAs1DForOutWhenUnconnected=off
  dwb : Outport  Port=10  PortDimensions=[3,1]  VectorParamsAs1DForOutWhenUnconnected=off
  wires:
  Reshape/1 -> "vb "/1
  f/1 -> 6DOF (Quaternion)/1
  tao/1 -> 6DOF (Quaternion)/2
  6DOF (Quaternion)/2 -> "xe "/1
  6DOF (Quaternion)/1 -> ve/1
  6DOF (Quaternion)/3 -> Euler/1
  Transpose/1 -> DCM/1
  6DOF (Quaternion)/5 -> Reshape/1
  6DOF (Quaternion)/6 -> "p,q,r "/1
  6DOF (Quaternion)/7 -> dwb/1
  6DOF (Quaternion)/8 -> Ab/1
  Direction Cosine Matrix to Quaternions/1 -> Quaternion/1
  6DOF (Quaternion)/9 -> Abe/1
  6DOF (Quaternion)/4 -> Transpose/1, Direction Cosine Matrix to Quaternions/1

== system LW_noaileron_dynamic/Rigid Model/WSH ==
  f : Inport
  tao : Inport  Port=2
  6DOF (Quaternion) : Subsystem
  "xe " : Outport  VectorParamsAs1DForOutWhenUnconnected=off
  ve : Outport  Port=2  VectorParamsAs1DForOutWhenUnconnected=off
  "p,q,r " : Outport  Port=3  VectorParamsAs1DForOutWhenUnconnected=off
  "vb " : Outport  Port=4  VectorParamsAs1DForOutWhenUnconnected=off
  DCM : Outport  Port=5  VectorParamsAs1DForOutWhenUnconnected=off
  Euler : Outport  Port=6  VectorParamsAs1DForOutWhenUnconnected=off
  Quaternion : Outport  Port=7  VectorParamsAs1DForOutWhenUnconnected=off
  Ab : Outport  Port=8  VectorParamsAs1DForOutWhenUnconnected=off
  Abe : Outport  Port=9  VectorParamsAs1DForOutWhenUnconnected=off
  dwb : Outport  Port=10  VectorParamsAs1DForOutWhenUnconnected=off
  wires:
  6DOF (Quaternion)/5(DCM) -> DCM/1
  6DOF (Quaternion)/6(Euler) -> Euler/1
  6DOF (Quaternion)/3("p,q,r ") -> "p,q,r "/1
  6DOF (Quaternion)/2(ve) -> ve/1
  6DOF (Quaternion)/1("xe ") -> "xe "/1
  6DOF (Quaternion)/4("vb ") -> "vb "/1
  6DOF (Quaternion)/7(Quaternion) -> Quaternion/1
  6DOF (Quaternion)/8(Ab) -> Ab/1
  6DOF (Quaternion)/9(Abe) -> Abe/1
  6DOF (Quaternion)/10(dwb) -> dwb/1
  tao/1 -> 6DOF (Quaternion)/2(tao)
  f/1 -> 6DOF (Quaternion)/1(f)

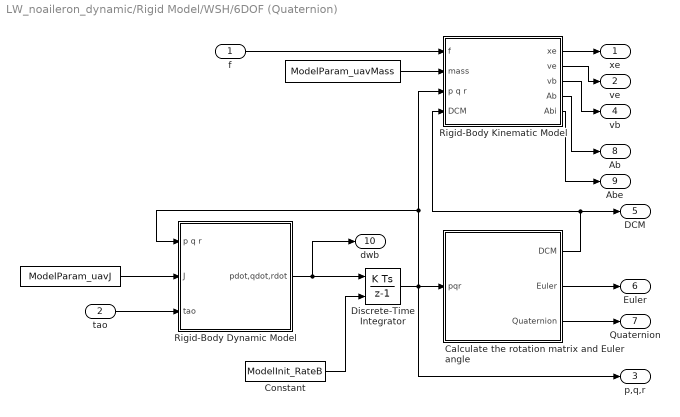
== system LW_noaileron_dynamic/Rigid Model/WSH/6DOF (Quaternion) ==
  f : Inport
  tao : Inport  Port=2
  " " : Constant  Value=ModelParam_uavJ
  "  " : Constant  Value=ModelParam_uavMass
  Calculate the rotation matrix and Euler angle : Subsystem
  Constant : Constant  Value=ModelInit_RateB
  Discrete-Time Integrator : DiscreteIntegrator  InitialConditionSource=external  SampleTime=-1  ICPrevOutput=DiscIntNeverNeededParam  ICPrevScaledInput=DiscIntNeverNeededParam
  Rigid-Body Dynamic Model : Subsystem
  Rigid-Body Kinematic Model : Subsystem
  "xe " : Outport  VectorParamsAs1DForOutWhenUnconnected=off
  ve : Outport  Port=2  VectorParamsAs1DForOutWhenUnconnected=off
  "p,q,r " : Outport  Port=3  VectorParamsAs1DForOutWhenUnconnected=off
  "vb " : Outport  Port=4  VectorParamsAs1DForOutWhenUnconnected=off
  DCM : Outport  Port=5  VectorParamsAs1DForOutWhenUnconnected=off
  Euler : Outport  Port=6  VectorParamsAs1DForOutWhenUnconnected=off
  Quaternion : Outport  Port=7  VectorParamsAs1DForOutWhenUnconnected=off
  Ab : Outport  Port=8  VectorParamsAs1DForOutWhenUnconnected=off
  Abe : Outport  Port=9  VectorParamsAs1DForOutWhenUnconnected=off
  dwb : Outport  Port=10  VectorParamsAs1DForOutWhenUnconnected=off
  wires:
  tao/1 -> Rigid-Body Dynamic Model/3(tao)
  Rigid-Body Kinematic Model/1("xe ") -> "xe "/1
  Constant/1 -> Discrete-Time Integrator/2
  Calculate the rotation matrix and Euler angle/1(DCM) -> DCM/1, Rigid-Body Kinematic Model/4(DCM)
  " "/1 -> Rigid-Body Dynamic Model/2(J)
  Rigid-Body Dynamic Model/1(pdot,qdot,rdot) -> dwb/1, Discrete-Time Integrator/1
  "  "/1 -> Rigid-Body Kinematic Model/2(mass)
  Rigid-Body Kinematic Model/2(ve) -> ve/1
  Calculate the rotation matrix and Euler angle/2(Euler) -> Euler/1
  f/1 -> Rigid-Body Kinematic Model/1(f)
  Discrete-Time Integrator/1 -> "p,q,r "/1, Rigid-Body Kinematic Model/3(p q r), Rigid-Body Dynamic Model/1(p q r), Calculate the rotation matrix and Euler angle/1(pqr)
  Rigid-Body Kinematic Model/3("vb ") -> "vb "/1
  Calculate the rotation matrix and Euler angle/3(Quaternion) -> Quaternion/1
  Rigid-Body Kinematic Model/4(Ab) -> Ab/1
  Rigid-Body Kinematic Model/5(Abi) -> Abe/1

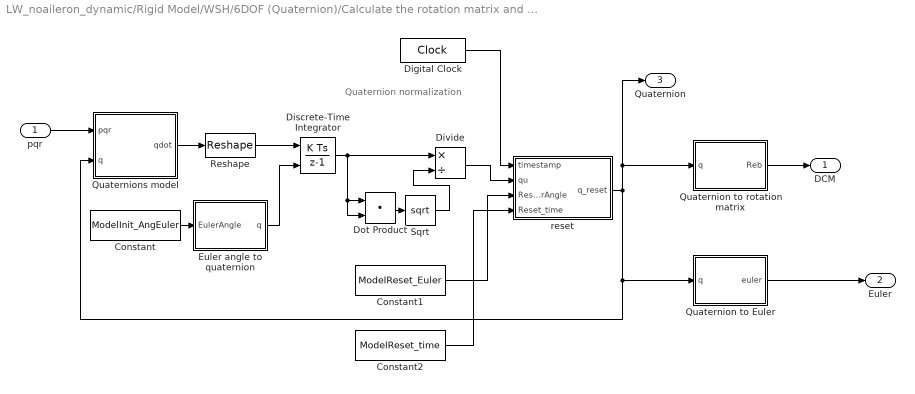
== system LW_noaileron_dynamic/Rigid Model/WSH/6DOF (Quaternion)/Calculate the rotation matrix and Euler angle ==
  note: Quaternion
      | normalization
  pqr : Inport
  Constant : Constant  Value=ModelInit_AngEuler
  Constant1 : Constant  Value=ModelReset_Euler  VectorParams1D=off
  Constant2 : Constant  Value=ModelReset_time
  Digital Clock : DigitalClock  SampleTime=0.001
  Discrete-Time Integrator : DiscreteIntegrator  InitialConditionSource=external  SampleTime=-1  ICPrevOutput=DiscIntNeverNeededParam  ICPrevScaledInput=DiscIntNeverNeededParam
  Divide : Product  Inputs=*/
  Dot Product : DotProduct  OutDataTypeStr=Inherit: Inherit via internal rule
  Euler angle to quaternion : MATLAB Function
  Quaternion to Euler : MATLAB Function
  Quaternion to rotation matrix : MATLAB Function
  Quaternions model : MATLAB Function  TreatAsAtomicUnit=on
  Reshape : Reshape  OutputDimensionality=Customize  OutputDimensions=[4,1]
  Sqrt : Sqrt
  reset : MATLAB Function
  DCM : Outport  VectorParamsAs1DForOutWhenUnconnected=off
  Euler : Outport  Port=2  VectorParamsAs1DForOutWhenUnconnected=off
  Quaternion : Outport  Port=3  VectorParamsAs1DForOutWhenUnconnected=off
  wires:
  Constant2/1 -> reset/4(Reset_time)
  Digital Clock/1 -> reset/1(timestamp)
  Constant1/1 -> reset/3(ResetEulerAngle)
  Divide/1 -> reset/2(qu)
  Reshape/1 -> Discrete-Time Integrator/1
  Euler angle to quaternion/1(q) -> Discrete-Time Integrator/2
  Constant/1 -> Euler angle to quaternion/1(EulerAngle)
  Quaternion to Euler/1(euler) -> Euler/1
  Quaternion to rotation matrix/1(Reb) -> DCM/1
  Quaternions model/1(qdot) -> Reshape/1
  Discrete-Time Integrator/1 -> Divide/1, Dot Product/2, Dot Product/1
  pqr/1 -> Quaternions model/1(pqr)
  Dot Product/1 -> Sqrt/1
  reset/1(q_reset) -> Quaternion to Euler/1(q), Quaternions model/2(q), Quaternion to rotation matrix/1(q), Quaternion/1
  Sqrt/1 -> Divide/2

== system LW_noaileron_dynamic/Rigid Model/WSH/6DOF (Quaternion)/Rigid-Body Dynamic Model ==
  p q r : Inport
  J : Inport  Port=2
  tao : Inport  Port=3
  Constant : Constant  Value=eye(3)
  Divide : Product  Inputs=*/  Multiplication=Matrix(*)
  J*w : Subsystem
  Product : Product  Multiplication=Matrix(*)
  Reshape : Reshape  OutputDimensionality=Customize  OutputDimensions=[3,1]
  Reshape1 : Reshape  OutputDimensionality=Column vector (2-D)
  Sum2 : Sum  Inputs=|+-
  wx(Jw) : sharedutil/3x3 Cross Product  aMode=aMode
  pdot,qdot,rdot : Outport  VectorParamsAs1DForOutWhenUnconnected=off
  wires:
  Reshape/1 -> pdot,qdot,rdot/1
  wx(Jw)/1 -> Sum2/2
  tao/1 -> Sum2/1
  J*w/1("J*w ") -> wx(Jw)/2
  p q r/1 -> wx(Jw)/1, J*w/1(p q r)
  J/1 -> J*w/2(J), Divide/2
  Sum2/1 -> Reshape1/1
  Divide/1 -> Product/1
  Constant/1 -> Divide/1
  Reshape1/1 -> Product/2
  Product/1 -> Reshape/1

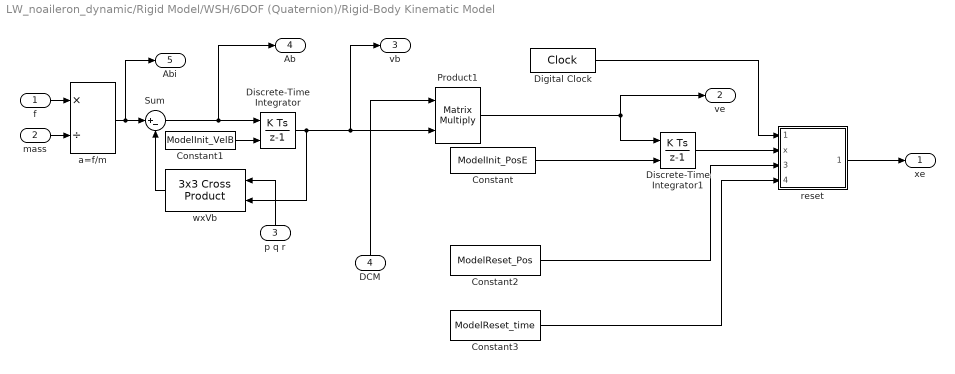
== system LW_noaileron_dynamic/Rigid Model/WSH/6DOF (Quaternion)/Rigid-Body Kinematic Model ==
  f : Inport
  mass : Inport  Port=2
  p q r : Inport  Port=3
  DCM : Inport  Port=4
  Constant : Constant  Value=ModelInit_PosE
  Constant1 : Constant  Value=ModelInit_VelB
  Constant2 : Constant  Value=ModelReset_Pos
  Constant3 : Constant  Value=ModelReset_time
  Digital Clock : DigitalClock  SampleTime=0.001
  Discrete-Time Integrator : DiscreteIntegrator  InitialConditionSource=external  SampleTime=-1  ICPrevOutput=DiscIntNeverNeededParam  ICPrevScaledInput=DiscIntNeverNeededParam
  Discrete-Time Integrator1 : DiscreteIntegrator  InitialConditionSource=external  SampleTime=-1  ICPrevOutput=DiscIntNeverNeededParam  ICPrevScaledInput=DiscIntNeverNeededParam
  Product1 : Product  Multiplication=Matrix(*)
  Sum : Sum  Inputs=|+-
  a=f/m : Product  Inputs=*/
  reset : MATLAB Function
  wxVb : sharedutil/3x3 Cross Product  aMode=aMode
  "xe " : Outport  VectorParamsAs1DForOutWhenUnconnected=off
  ve : Outport  Port=2  VectorParamsAs1DForOutWhenUnconnected=off
  "vb " : Outport  Port=3  VectorParamsAs1DForOutWhenUnconnected=off
  Ab : Outport  Port=4  VectorParamsAs1DForOutWhenUnconnected=off
  Abi : Outport  Port=5  VectorParamsAs1DForOutWhenUnconnected=off
  wires:
  Discrete-Time Integrator1/1 -> reset/2(x)
  Constant3/1 -> reset/4(Reset_time)
  Constant2/1 -> reset/3(ResetPos)
  Digital Clock/1 -> reset/1(timestamp)
  wxVb/1 -> Sum/2
  Constant1/1 -> Discrete-Time Integrator/2
  Constant/1 -> Discrete-Time Integrator1/2
  p q r/1 -> wxVb/1
  f/1 -> a=f/m/1
  mass/1 -> a=f/m/2
  DCM/1 -> Product1/1
  Product1/1 -> Discrete-Time Integrator1/1, ve/1
  reset/1(x_reset) -> "xe "/1
  Sum/1 -> Ab/1, Discrete-Time Integrator/1
  a=f/m/1 -> Abi/1, Sum/1
  Discrete-Time Integrator/1 -> wxVb/2, "vb "/1, Product1/2

== system LW_noaileron_dynamic/Rigid Model/WSH/6DOF (Quaternion)/Rigid-Body Dynamic Model/J*w ==
  p q r : Inport
  J : Inport  Port=2
  J*w : Product  Multiplication=Matrix(*)
  "J*w " : Outport  VectorParamsAs1DForOutWhenUnconnected=off
  wires:
  p q r/1 -> J*w/2
  J/1 -> J*w/1
  J*w/1 -> "J*w "/1

== matlab function LW_noaileron_dynamic/Rigid Model/WSH/6DOF (Quaternion)/Calculate the rotation matrix and Euler angle/reset ==
  data: timestamp input; qu input; q_reset output; ResetEulerAngle input; Reset_time input
function q_reset = fcn(timestamp, qu, ResetEulerAngle, Reset_time)

resetNum = 0;
resetTotalNum = length(Reset_time);
if ~isempty(Reset_time)
    for i=1:resetTotalNum
        if resetTotalNum < 1.5
            if timestamp >= Reset_time(1)
                resetNum = 1;
                break;
            end
        else
            if i>=resetTotalNum
                if timestamp >= Reset_time(i)
                    resetNum = i;
                    break;
                end
            else
                if timestamp >= Reset_time(i) && timestamp < Reset_time(i+1)
                    resetNum = i;
                    break;
                end
            end
        end
    end
    if resetNum >0
        ResetEuler = sum(ResetEulerAngle(1:resetNum,1:3),1);%积分的初始值没变，所以这里需要累加
        q_delta = eul2quat([ResetEuler(3) ResetEuler(2) ResetEuler(1)],'ZYX');
        q_reset_num = quatmultiply(q_delta,qu');
        q_reset = q_reset_num';
    else
        q_reset = qu;
    end
else
    q_reset = qu;
end

== matlab function LW_noaileron_dynamic/Rigid Model/WSH/6DOF (Quaternion)/Rigid-Body Kinematic Model/reset ==
  data: timestamp input; x input; x_reset output; ResetPos input; Reset_time input
function x_reset = fcn(timestamp, x, ResetPos, Reset_time)
%Function description:
%  Get quaternions from Euler angle

resetNum = 0;
resetTotalNum = length(Reset_time);
if ~isempty(Reset_time)
    for i=1:resetTotalNum
        if resetTotalNum < 1.5
            if timestamp >= Reset_time(1)
                resetNum = 1;
                break;
            end
        else
            if i>=resetTotalNum
                if timestamp >= Reset_time(i)
                    resetNum = i;
                    break;
                end
            else
                if timestamp >= Reset_time(i) && timestamp < Reset_time(i+1)
                    resetNum = i;
                    break;
                end
            end
        end
    end
    if resetNum >0
        x_reset = x(:) + sum(ResetPos(1:resetNum,1:3),1)';
    else
        x_reset = x(:);
    end
else
    x_reset = x(:);
end
% if timestamp >= Reset_time
%     x_reset = x + ResetPos;
% else
%     x_reset = x;
% end

== matlab function LW_noaileron_dynamic/Forces and Moments/b2l ==
  data: F input; Fa_l output; LW_ANGLE parameter
function Fa_l  = fcn(F, LW_ANGLE)
k = LW_ANGLE*pi/180;
Rm = [cos(k), 0 , -sin(k);
    0,     1 ,    0;
    sin(k), 0 ,  cos(k)];
Fa_l = Rm*F;

== matlab function LW_noaileron_dynamic/Environment Models/Ground Model ==
  settings: updateMethod=DISCRETE
  data: terrainZ input; Ve input; Xe input; landed output; takeoff output
function [landed,takeoff] = fcn(terrainZ, Ve, Xe)
% This is a ground model that can provides reaction force and reaction torque

persistent takeoffFlag;
if isempty(takeoffFlag)
     takeoffFlag=int8(0);
end

persistent landFlag;
if isempty(landFlag)
     landFlag=int8(1);
end


z=Xe(3)-terrainZ;

 if ((z < -0.001) && (Ve(3)<-0.01)|| z < 1.0) && (takeoffFlag < 0.5)
    takeoffFlag = int8(1);
    landFlag = int8(0);
 end
 
 if (z>-0.00001)&&(landFlag<0.5)
    landFlag=int8(1);
    takeoffFlag=int8(0);
    %z0=terrainZ;
 end

takeoff = takeoffFlag;
landed = landFlag;

end

== matlab function LW_noaileron_dynamic/Forces and Moments/b2l1 ==
  data: Ma input; Ma_l output; LW_ANGLE parameter
function Ma_l  = fcn(Ma, LW_ANGLE)
kk = LW_ANGLE*pi/180;
Rm = [cos(kk), 0 , -sin(kk);
    0,     1 ,    0;
    sin(kk), 0 ,  cos(kk)];
Ma_l = Rm*Ma;
